simulink model "sixDOFTest"  (R2023a)
settings: Solver=VariableStepAuto  StartTime=0.0  StopTime=30  RelTol=1e-3
libraries: shared6dof x1, aerolibanim x1
settings Model: Creator=ericyang  LastModifiedBy=ericyang

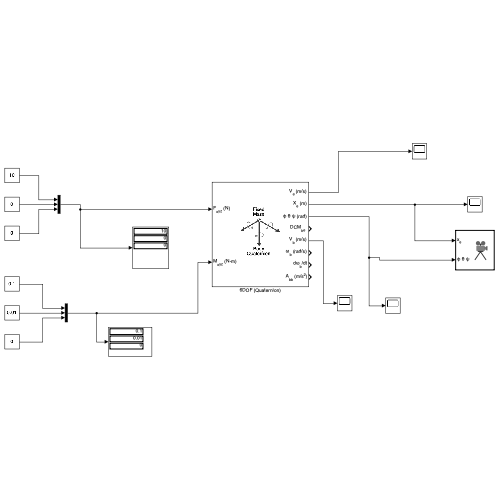
[thumbnail: Simulink's stored preview of the top-level diagram]
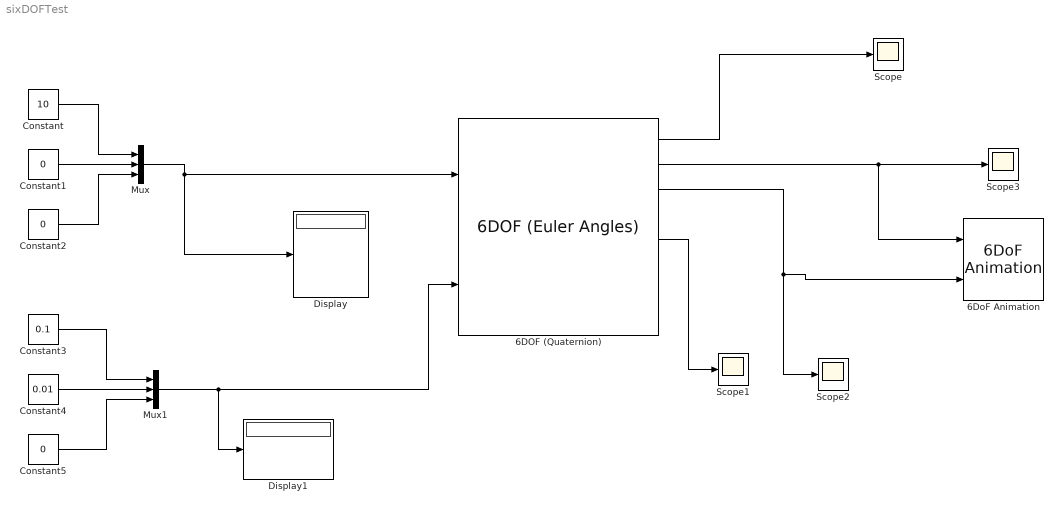
== system sixDOFTest ==
  6DOF (Quaternion) : shared6dof/6DOF (Euler Angles)  units=Metric (MKS)  mtype=Fixed  rep=Quaternion  xme_0=[0 0 0]  Vm_0=[0 0 0]  eul_0=[0 pi/2 0]  pm_0=[0 0 0]  mass_0=1.0  mass_e=0.5  mass_f=2.0  inertia=eye(3)  inertia_e=eye(3)  inertia_f=2*eye(3)  k_quat=1.0  vre_flag=on  abi_flag=off  aMode=0  xme_statename=''  Vm_statename=''  eul_statename=''  quat_statename=''  pm_statename=''  mass_statename=''
      settings: LibrarySourceBlock=aerolib6dof2/6DOF (Quaternion)
  6DoF Animation : aerolibanim/6DoF Animation  u1=[0 2000 0 2000 -5000 0]  u2=0.1  u3=1000  u4=[-100000, 0, 0]  u5=Fixed position  u6=[5000 7000 -8000]  u7=0  u8=on
  Constant : Constant  Value=10
  Constant1 : Constant  Value=0
  Constant2 : Constant  Value=0
  Constant3 : Constant  Value=0.1
  Constant4 : Constant  Value=0.01
  Constant5 : Constant  Value=0
  Display : Display
  Display1 : Display
  Mux : Mux  Inputs=3
  Mux1 : Mux  Inputs=3
  Scope{,1..3} (4 alike) : Scope
  wires:
  Constant/1 -> Mux/1
  Constant1/1 -> Mux/2
  Constant2/1 -> Mux/3
  Constant3/1 -> Mux1/1
  Constant4/1 -> Mux1/2
  Constant5/1 -> Mux1/3
  Mux1/1 -> 6DOF (Quaternion)/2, Display1/1
  Mux/1 -> 6DOF (Quaternion)/1, Display/1
  6DOF (Quaternion)/2 -> 6DoF Animation/1, Scope3/1
  6DOF (Quaternion)/3 -> Scope2/1, 6DoF Animation/2
  6DOF (Quaternion)/1 -> Scope/1
  6DOF (Quaternion)/5 -> Scope1/1
